simulink model "VelRefControlSim_ForThesis"  (R2016b)
settings: Solver=ode2  StartTime=0.0  StopTime=525  FixedStep=0.001  MaxStep=0.01  MinStep=0.0005  RelTol=1e-2  AbsTol=1e-3
undefined symbols (not defined in the file or in its folder): DiscIntNeverNeededParam, model_identific_dy8147ea57gM
libraries: simulink x8, powerlib_meascontrol x3, dspswit3 x1, fmu_cs_lib x1
settings Model: Creator=vamsikrishna95  LastModifiedBy=vamsikrishna95
settings SolverCC: InitialStep=0.0005  MaxConsecutiveMinStep=100  ZeroCrossAlgorithm=Adaptive

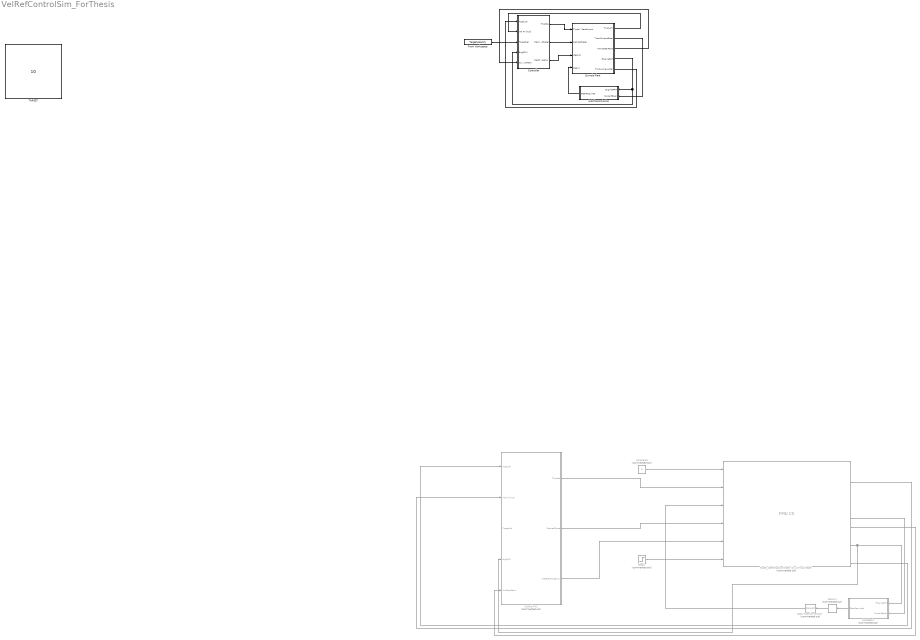
== system VelRefControlSim_ForThesis ==
  AutoGear1 : Subsystem  Commented=on
  AutoTransmission : Subsystem
  Constant1 : Constant  Commented=on  Value=0  OutDataTypeStr=Inherit: Inherit via back propagation
  Control FV2 : Subsystem  Commented=on
  Controller : Subsystem
  Data Type Conversion : DataTypeConversion  Commented=on
  Dymola Plant : Subsystem  Tag=21-Aug-2018 15:18:52#8147  LoadFcn=if exist('newDymolaGui') newDymolaGui('VelRefControlSim_TemptoDel/Dymola Plant','PostLoadNew'); else error('Dymola not installed. Must install at least the file newDymolaGui.p'); end;
      mask help:
      | Dymola block.
      | A dymola block allows acausal physical modeling.
      | See Dymola manual for usage.
      settings: CopyFcn=newDymolaGui('21-Aug-2018 15:18:52#8147','Copy');  DeleteFcn=if exist('newDymolaGui') newDymolaGui('VelRefControlSim_TemptoDel/Dymola Plant','Delete'); end;  NameChangeFcn=newDymolaGui('21-Aug-2018 15:18:52#8147','Copy');  OpenFcn=newDymolaGui('VelRefControlSim_TemptoDel/Dymola Plant','Init');
  From Workspace : FromWorkspace  VariableName=TargetVelocity  SampleTime=0
  Memory : Memory  Commented=on  X0=2  InheritSampleTime=on
  Model_Identification.Model_ID_v2.TruckModel : fmu_cs_lib/FMU CS  Description=Simulates an FMU for Co-Simulation 1.0 or Co-Simulation 2.0.  Commented=on  dummy=0
  Step1 : Step  Commented=on  Time=3  Before=1  After=0  SampleTime=0
  TARGET : Constant  Value=10  OutDataTypeStr=Inherit: Inherit via back propagation
  wires:
  AutoGear1/1(GearRequired) -> Memory/1
  Model_Identification.Model_ID_v2.TruckModel/7 -> AutoGear1/2(CurrentGear)
  Model_Identification.Model_ID_v2.TruckModel/10 -> Control FV2/4(EngRPM), AutoGear1/1(EngineRPM)
  Memory/1 -> Data Type Conversion/1
  Data Type Conversion/1 -> Model_Identification.Model_ID_v2.TruckModel/3
  Step1/1 -> Model_Identification.Model_ID_v2.TruckModel/6
  Constant1/1 -> Model_Identification.Model_ID_v2.TruckModel/1
  Controller/1(Throttle) -> Dymola Plant/1(ThrottlePedalInput)
  Controller/2(DesiredDecel) -> Dymola Plant/2(DesiredDecel)
  Controller/3(DesBrakeUrgency) -> Dymola Plant/3(Urgency)
  Control FV2/1(Throttle) -> Model_Identification.Model_ID_v2.TruckModel/2
  Control FV2/2(DesiredDecel) -> Model_Identification.Model_ID_v2.TruckModel/4
  Control FV2/3(DesBrakeUrgency) -> Model_Identification.Model_ID_v2.TruckModel/5
  Model_Identification.Model_ID_v2.TruckModel/12 -> Control FV2/1(Accel_FV)
  Model_Identification.Model_ID_v2.TruckModel/3 -> Control FV2/2(Vel FV [m/s])
  Model_Identification.Model_ID_v2.TruckModel/8 -> Control FV2/5(CurGearRatio)
  Dymola Plant/2(TransCurrentGear) -> AutoTransmission/2(CurrentGear)
  Dymola Plant/5(Truck_Long_Accel) -> Controller/1(Accel_FV)
  Dymola Plant/4(EngineRPM) -> Controller/4(EngRPM), AutoTransmission/1(EngineRPM)
  Dymola Plant/3(TransGearRatio) -> Controller/5(CurGearRatio)
  Dymola Plant/1(Truck_dX) -> Controller/2(Vel FV [m/s])
  AutoTransmission/1(GearRequired) -> Dymola Plant/4(GearIn)
  From Workspace/1 -> Controller/3(TargetVel)

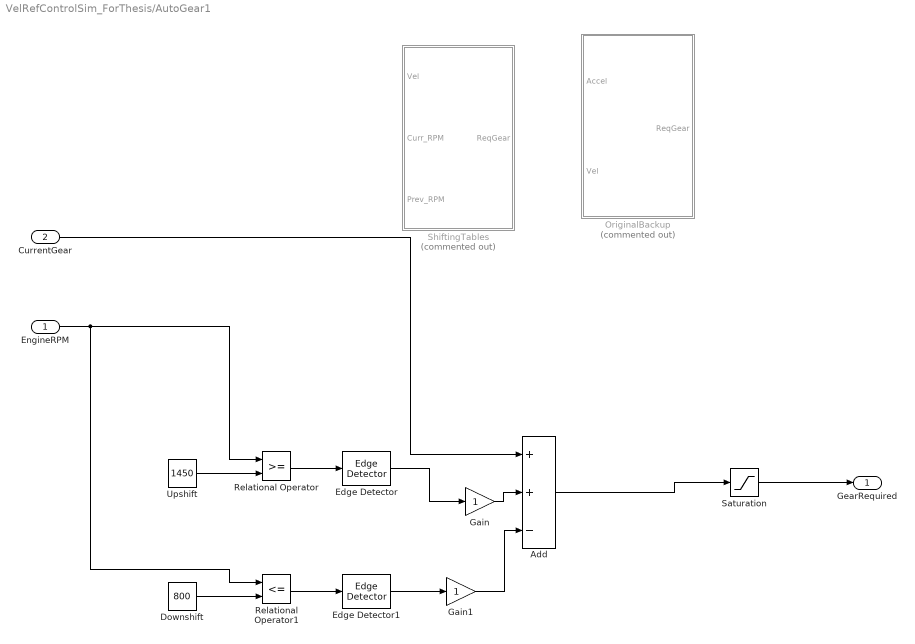
== system VelRefControlSim_ForThesis/AutoGear1 ==
  EngineRPM : Inport
  CurrentGear : Inport  Port=2
  Add : Sum  Inputs=++-
  Downshift : Constant  Value=800
  Edge Detector : powerlib_meascontrol/Logic/Edge Detector  model=Rising  ic=0  Ts=0
  Edge Detector1 : powerlib_meascontrol/Logic/Edge Detector  model=Rising  ic=0  Ts=0
  Gain : Gain
  Gain1 : Gain
  OriginalBackup : MATLAB Function  Commented=on  TreatAsAtomicUnit=on
  Relational Operator : RelationalOperator  OutDataTypeStr=boolean  RndMeth=Simplest
  Relational Operator1 : RelationalOperator  Operator=<=  OutDataTypeStr=boolean  RndMeth=Simplest
  Saturation : Saturate  UpperLimit=10  LowerLimit=0
  ShiftingTables : MATLAB Function  Commented=on  TreatAsAtomicUnit=on
  Upshift : Constant  Value=1450
  GearRequired : Outport
  wires:
  EngineRPM/1 -> Relational Operator1/1, Relational Operator/1
  Upshift/1 -> Relational Operator/2
  Downshift/1 -> Relational Operator1/2
  Relational Operator/1 -> Edge Detector/1
  Relational Operator1/1 -> Edge Detector1/1
  CurrentGear/1 -> Add/1
  Add/1 -> Saturation/1
  Edge Detector/1 -> Gain/1
  Gain/1 -> Add/2
  Edge Detector1/1 -> Gain1/1
  Gain1/1 -> Add/3
  Saturation/1 -> GearRequired/1

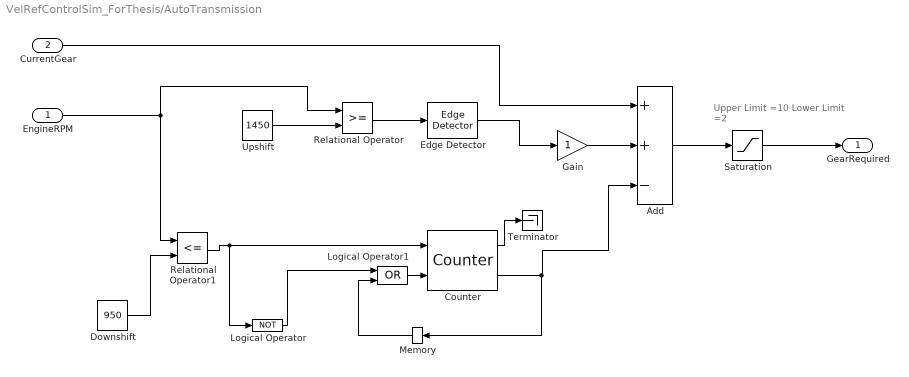
== system VelRefControlSim_ForThesis/AutoTransmission ==
  note: Upper Limit =10
      | Lower Limit =2
  EngineRPM : Inport
  CurrentGear : Inport  Port=2
  Add : Sum  Inputs=++-
  Counter : dspswit3/Counter  Direction=Up  CountEvent=Non-zero sample  CounterSize=32 bits  MaxCount=250  InitialCount=0  Output=Count and Hit  HitValue=500  ResetInput=on  SamplesPerFrame=1  Ts=1  CntDtype=double  HitDtype=Boolean
  Downshift : Constant  Value=950
  Edge Detector : powerlib_meascontrol/Logic/Edge Detector  model=Rising  ic=0  Ts=0
  Gain : Gain
  Logical Operator : Logic  Operator=NOT  AllPortsSameDT=off  OutDataTypeStr=boolean
  Logical Operator1 : Logic  Operator=OR  AllPortsSameDT=off  OutDataTypeStr=boolean
  Memory : Memory
  Relational Operator : RelationalOperator  OutDataTypeStr=boolean  RndMeth=Simplest
  Relational Operator1 : RelationalOperator  Operator=<=  OutDataTypeStr=boolean  RndMeth=Simplest
  Saturation : Saturate  UpperLimit=10  LowerLimit=2
  Terminator : Terminator
  Upshift : Constant  Value=1450
  GearRequired : Outport
  wires:
  EngineRPM/1 -> Relational Operator/1, Relational Operator1/1
  Upshift/1 -> Relational Operator/2
  Downshift/1 -> Relational Operator1/2
  Relational Operator/1 -> Edge Detector/1
  Relational Operator1/1 -> Logical Operator/1, Counter/1
  CurrentGear/1 -> Add/1
  Add/1 -> Saturation/1
  Edge Detector/1 -> Gain/1
  Gain/1 -> Add/2
  Counter/2 -> Add/3, Memory/1
  Saturation/1 -> GearRequired/1
  Logical Operator/1 -> Logical Operator1/1
  Logical Operator1/1 -> Counter/2
  Memory/1 -> Logical Operator1/2
  Counter/1 -> Terminator/1

== system VelRefControlSim_ForThesis/Control FV2 ==
  Accel_FV : Inport
  Vel FV [m/s] : Inport  Port=2
  TargetVel : Inport  Port=3
  EngRPM : Inport  Port=4
  CurGearRatio : Inport  Port=5
  TAMU_LC3 : Subsystem
  Throttle : Outport
  DesiredDecel : Outport  Port=2
  DesBrakeUrgency : Outport  Port=3
  wires:
  EngRPM/1 -> TAMU_LC3/5(EngRPM1)
  Accel_FV/1 -> TAMU_LC3/1(aFV_mps2)
  TAMU_LC3/1(Throttle) -> Throttle/1
  TAMU_LC3/2(DesiredDecel) -> DesiredDecel/1
  TAMU_LC3/3(DesBrakeUrgency) -> DesBrakeUrgency/1
  CurGearRatio/1 -> TAMU_LC3/3(CurGearRatio)
  TargetVel/1 -> TAMU_LC3/4(TargetVel)
  Vel FV [m/s]/1 -> TAMU_LC3/2(vFV_mps)

== system VelRefControlSim_ForThesis/Controller ==
  Accel_FV : Inport
  Vel FV [m/s] : Inport  Port=2
  TargetVel : Inport  Port=3
  EngRPM : Inport  Port=4
  CurGearRatio : Inport  Port=5
  TAMU_LC3 : Subsystem
  Throttle : Outport
  DesiredDecel : Outport  Port=2
  DesBrakeUrgency : Outport  Port=3
  wires:
  Vel FV [m/s]/1 -> TAMU_LC3/2(Current_Velocity)
  TargetVel/1 -> TAMU_LC3/4(Target_Velocity)
  CurGearRatio/1 -> TAMU_LC3/3(CurGearRatio)
  TAMU_LC3/3(DesBrakeUrgency) -> DesBrakeUrgency/1
  TAMU_LC3/2(DesiredDeceleration) -> DesiredDecel/1
  TAMU_LC3/1(Throttle) -> Throttle/1
  Accel_FV/1 -> TAMU_LC3/1(Current_Acceleration)
  EngRPM/1 -> TAMU_LC3/5(EngineRPM)

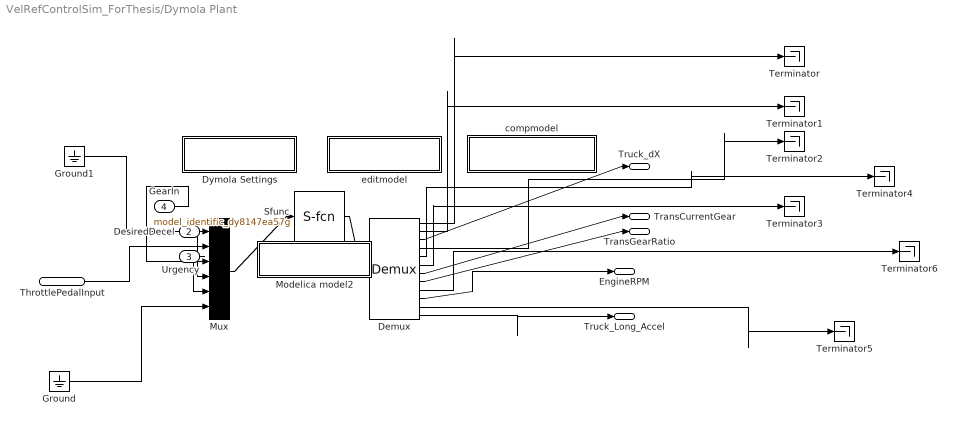
== system VelRefControlSim_ForThesis/Dymola Plant ==
  ThrottlePedalInput : Inport
  DesiredDecel : Inport  Port=2
  Urgency : Inport  Port=3
  GearIn : Inport  Port=4
  Demux : Demux  Outputs=[1;1;1;1;1;1;1;1;1;1;1;1]
  Dymola Settings : Subsystem  mask{ModelName=Model_Identification.Model_ID_v2.TruckModel, MoFileName=C:/Users/vamsikrishna95/OneDrive - Texas A&M University/MS Research/Dymola/Model Identification/Model_Identification.mo, dSpace=, BusConnector=[], ResultFile=[], ResultFileOnline=[], ResultDt=[], Libs=:HydraulicsLib:, bigobj=1, ImportFolder=[], guimode=[], ModelName2=[], forRuntime=[], MEXLoad=[], omitDescription=[]}
      mask prompts: ModelName "Name of Dymola model"; MoFileName "File Name (including .mo)"; ResultFile "Create Result"; ResultFileOnline "Load result"; ResultDt "Result min dt"; Libs "Used Libraries"; bigobj "Compiler flag /bigobj"; ImportFolder "Import folder"; guimode "GUI mode flag"; ModelName2 "Model name for import mode"; forRuntime "Runtime export"; MEXLoad "Compiled S-function"; omitDescription "Omit description strings"
      mask Display: disp('Dymola Settings');
  Ground : Ground
  Ground1 : Ground
  Modelica model2 : Subsystem
      mask Display: disp('Change parameters');
  Mux : Mux  Inputs=[1;1;1;1;1;1]
  Sfunc : S-Function  Tag=8147ea57g  FunctionName=model_identific_dy8147ea57g  Parameters=[model_identific_dy8147ea57gM.pV],[model_identific_dy8147ea57gM.x0V]  PortCounts=[1;1]  SFunctionDeploymentMode=off  EnableBusSupport=off
      mask Display: image(imread('Dymola.bmp'))
  Terminator{,1..6} (7 alike) : Terminator
  compmodel : Subsystem
      settings: OpenFcn=compileModelica('VelRefControlSim_TemptoDel/Dymola Plant');
      mask Display: disp('Compile Modelica model');
  editmodel : Subsystem
      settings: OpenFcn=editModelica('VelRefControlSim_TemptoDel/Dymola Plant');
      mask Display: disp('Edit Modelica model');
  Truck_dX : Outport
  TransCurrentGear : Outport  Port=2
  TransGearRatio : Outport  Port=3
  EngineRPM : Outport  Port=4
  Truck_Long_Accel : Outport  Port=5
  wires:
  Sfunc/1 -> Demux/1
  Demux/1 -> Terminator/1
  Demux/2 -> Terminator1/1
  Demux/3 -> Truck_dX/1
  Demux/4 -> Terminator2/1
  Demux/5 -> Terminator4/1
  Demux/6 -> Terminator3/1
  Demux/7 -> TransCurrentGear/1
  Demux/8 -> TransGearRatio/1
  Demux/9 -> Terminator6/1
  Demux/10 -> EngineRPM/1
  Demux/11 -> Terminator5/1
  Demux/12 -> Truck_Long_Accel/1
  Mux/1 -> Sfunc/1
  Ground1/1 -> Mux/1
  ThrottlePedalInput/1 -> Mux/2
  GearIn/1 -> Mux/3
  DesiredDecel/1 -> Mux/4
  Urgency/1 -> Mux/5
  Ground/1 -> Mux/6

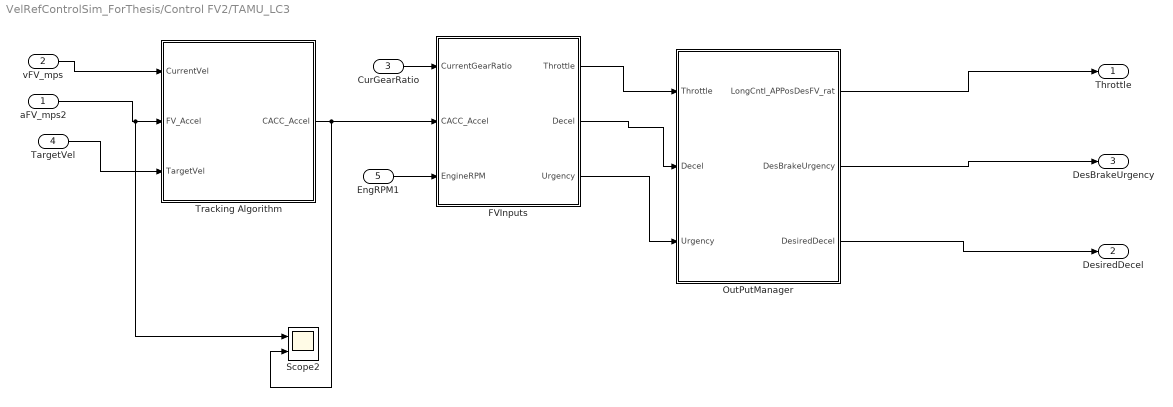
== system VelRefControlSim_ForThesis/Control FV2/TAMU_LC3 ==
  aFV_mps2 : Inport
  vFV_mps : Inport  Port=2
  CurGearRatio : Inport  Port=3
  TargetVel : Inport  Port=4
  EngRPM1 : Inport  Port=5
  FVInputs : Subsystem
  OutPutManager : Subsystem
  Scope2 : Scope  NumInputPorts=2
  Tracking Algorithm : Subsystem
  Throttle : Outport
  DesiredDecel : Outport  Port=2
  DesBrakeUrgency : Outport  Port=3
  wires:
  Tracking Algorithm/1(CACC_Accel) -> Scope2/2, FVInputs/2(CACC_Accel)
  vFV_mps/1 -> Tracking Algorithm/1(CurrentVel)
  EngRPM1/1 -> FVInputs/3(EngineRPM)
  CurGearRatio/1 -> FVInputs/1(CurrentGearRatio)
  aFV_mps2/1 -> Scope2/1, Tracking Algorithm/2(FV_Accel)
  FVInputs/1(Throttle) -> OutPutManager/1(Throttle)
  FVInputs/3(Urgency) -> OutPutManager/3(Urgency)
  OutPutManager/1(LongCntl_APPosDesFV_rat) -> Throttle/1
  OutPutManager/2(DesBrakeUrgency) -> DesBrakeUrgency/1
  OutPutManager/3(DesiredDecel) -> DesiredDecel/1
  FVInputs/2(Decel) -> OutPutManager/2(Decel)
  TargetVel/1 -> Tracking Algorithm/3(TargetVel)

== system VelRefControlSim_ForThesis/Controller/TAMU_LC3 ==
  Current_Acceleration : Inport
  Current_Velocity : Inport  Port=2
  CurGearRatio : Inport  Port=3
  Target_Velocity : Inport  Port=4
  EngineRPM : Inport  Port=5
  OutPutManager : Subsystem
  Plant Inversion : Subsystem
  Tracking Algorithm : Subsystem
  Throttle : Outport
  DesiredDeceleration : Outport  Port=2
  DesBrakeUrgency : Outport  Port=3
  wires:
  Tracking Algorithm/1(Target_Accel) -> Plant Inversion/3(Target_Accel)
  Current_Velocity/1 -> Plant Inversion/2(CurrentVelocity), Tracking Algorithm/1(CurrentVel)
  EngineRPM/1 -> Plant Inversion/4(EngineRPM)
  CurGearRatio/1 -> Plant Inversion/1(CurrentGearRatio)
  Current_Acceleration/1 -> Tracking Algorithm/2(FV_Accel)
  Plant Inversion/1(Throttle) -> OutPutManager/1(Throttle)
  Plant Inversion/3(Urgency) -> OutPutManager/3(Urgency)
  OutPutManager/1(ThrottlePosition) -> Throttle/1
  OutPutManager/2(DesBrakeUrgency) -> DesBrakeUrgency/1
  OutPutManager/3(DesiredDecel) -> DesiredDeceleration/1
  Plant Inversion/2(Decel) -> OutPutManager/2(Decel)
  Target_Velocity/1 -> Tracking Algorithm/3(TargetVel)

== system VelRefControlSim_ForThesis/Dymola Plant/Dymola Settings ==

== system VelRefControlSim_ForThesis/Dymola Plant/Modelica model2 ==

== system VelRefControlSim_ForThesis/Dymola Plant/compmodel ==

== system VelRefControlSim_ForThesis/Dymola Plant/editmodel ==

== system VelRefControlSim_ForThesis/Control FV2/TAMU_LC3/FVInputs ==
  CurrentGearRatio : Inport
  CACC_Accel : Inport  Port=2
  EngineRPM : Inport  Port=3
  CalculateCommands : Subsystem
  Vel1 : InportShadow
  Throttle : Outport
  Decel : Outport  Port=2
  Urgency : Outport  Port=3
  wires:
  CalculateCommands/1(Throttle) -> Throttle/1
  CalculateCommands/3(Urgency) -> Urgency/1
  CalculateCommands/2(Decel) -> Decel/1
  CACC_Accel/1 -> CalculateCommands/1(AccelerationCommand)
  Vel1/1 -> CalculateCommands/3(Vel)
  EngineRPM/1 -> CalculateCommands/4(CurrentRPM)
  CurrentGearRatio/1 -> CalculateCommands/2(GearRatio)

== system VelRefControlSim_ForThesis/Control FV2/TAMU_LC3/OutPutManager ==
  Throttle : Inport
  Decel : Inport  Port=2
  Urgency : Inport  Port=3
  LongCntl_APPosDesFV_rat : Outport
  DesBrakeUrgency : Outport  Port=2
  DesiredDecel : Outport  Port=3
  wires:
  Throttle/1 -> LongCntl_APPosDesFV_rat/1
  Urgency/1 -> DesBrakeUrgency/1
  Decel/1 -> DesiredDecel/1

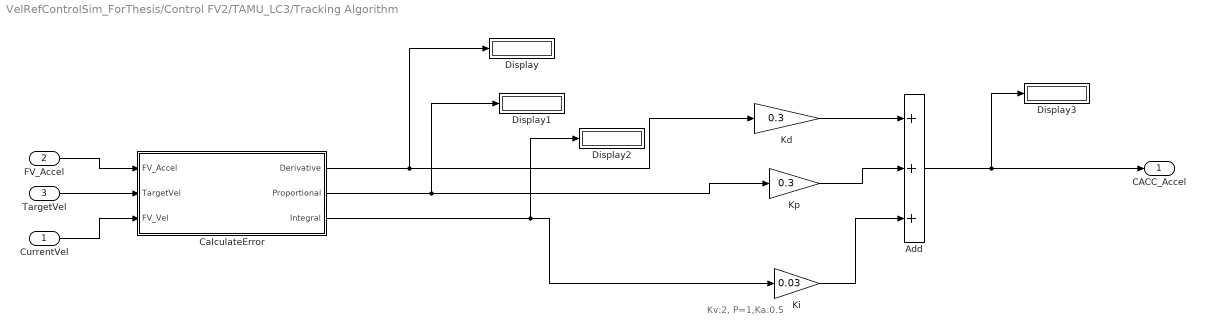
== system VelRefControlSim_ForThesis/Control FV2/TAMU_LC3/Tracking Algorithm ==
  note: Kv:2, P=1,Ka:0.5
  CurrentVel : Inport
  FV_Accel : Inport  Port=2
  TargetVel : Inport  Port=3
  Add : Sum  Inputs=+++
  CalculateError : Subsystem
  Display{,1..3} (4 alike) : Display
  Kd : Gain  Gain=0.3
  Ki : Gain  Gain=0.03
  Kp : Gain  Gain=0.3
  CACC_Accel : Outport
  wires:
  Add/1 -> Display3/1, CACC_Accel/1
  Ki/1 -> Add/3
  Kp/1 -> Add/2
  Kd/1 -> Add/1
  TargetVel/1 -> CalculateError/2(TargetVel)
  CalculateError/3(Integral) -> Display2/1, Ki/1
  CalculateError/1(Derivative) -> Display/1, Kd/1
  CalculateError/2(Proportional) -> Display1/1, Kp/1
  CurrentVel/1 -> CalculateError/3(FV_Vel)
  FV_Accel/1 -> CalculateError/1(FV_Accel)

== system VelRefControlSim_ForThesis/Controller/TAMU_LC3/OutPutManager ==
  Throttle : Inport
  Decel : Inport  Port=2
  Urgency : Inport  Port=3
  ThrottlePosition : Outport
  DesBrakeUrgency : Outport  Port=2
  DesiredDecel : Outport  Port=3
  wires:
  Throttle/1 -> ThrottlePosition/1
  Urgency/1 -> DesBrakeUrgency/1
  Decel/1 -> DesiredDecel/1

== system VelRefControlSim_ForThesis/Controller/TAMU_LC3/Plant Inversion ==
  CurrentGearRatio : Inport
  CurrentVelocity : Inport  Port=2
  Target_Accel : Inport  Port=3
  EngineRPM : Inport  Port=4
  CalculateCommands : Subsystem
  Throttle : Outport
  Decel : Outport  Port=2
  Urgency : Outport  Port=3
  wires:
  CalculateCommands/1(Throttle) -> Throttle/1
  CalculateCommands/3(Urgency) -> Urgency/1
  CalculateCommands/2(Decel) -> Decel/1
  Target_Accel/1 -> CalculateCommands/1(Target_Accel)
  CurrentVelocity/1 -> CalculateCommands/3(Vel)
  EngineRPM/1 -> CalculateCommands/4(CurrentRPM)
  CurrentGearRatio/1 -> CalculateCommands/2(GearRatio)

== system VelRefControlSim_ForThesis/Controller/TAMU_LC3/Tracking Algorithm ==
  CurrentVel : Inport
  FV_Accel : Inport  Port=2
  TargetVel : Inport  Port=3
  Add : Sum  Inputs=+++
  CalculateError : Subsystem
  Kd : Gain  Gain=0.3
  Ki : Gain  Gain=0.03
  Kp : Gain  Gain=1.5
  Target_Accel : Outport
  wires:
  Add/1 -> Target_Accel/1
  Ki/1 -> Add/3
  Kp/1 -> Add/2
  Kd/1 -> Add/1
  TargetVel/1 -> CalculateError/2(TargetVel)
  CalculateError/3(Integral) -> Ki/1
  CalculateError/1(Derivative) -> Kd/1
  CalculateError/2(Proportional) -> Kp/1
  CurrentVel/1 -> CalculateError/3(FV_Vel)
  FV_Accel/1 -> CalculateError/1(FV_Accel)

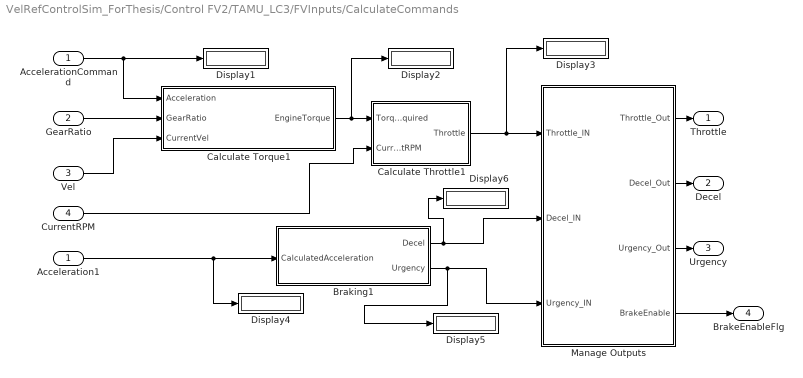
== system VelRefControlSim_ForThesis/Control FV2/TAMU_LC3/FVInputs/CalculateCommands ==
  AccelerationCommand : Inport
  GearRatio : Inport  Port=2
  Vel : Inport  Port=3
  CurrentRPM : Inport  Port=4
  Acceleration1 : InportShadow
  Braking1 : Subsystem
  Calculate Throttle1 : Subsystem
  Calculate Torque1 : Subsystem
  Display{1..6} (6 alike) : Display
  Manage Outputs : Subsystem
  Throttle : Outport
  Decel : Outport  Port=2
  Urgency : Outport  Port=3
  BrakeEnableFlg : Outport  Port=4
  wires:
  Vel/1 -> Calculate Torque1/3(CurrentVel)
  Manage Outputs/1(Throttle_Out) -> Throttle/1
  Manage Outputs/2(Decel_Out) -> Decel/1
  Manage Outputs/3(Urgency_Out) -> Urgency/1
  Manage Outputs/4(BrakeEnable) -> BrakeEnableFlg/1
  Calculate Torque1/1(EngineTorque) -> Display2/1, Calculate Throttle1/1(TorqueRequired)
  Braking1/1(Decel) -> Display6/1, Manage Outputs/2(Decel_IN)
  Braking1/2(Urgency) -> Display5/1, Manage Outputs/3(Urgency_IN)
  Calculate Throttle1/1(Throttle) -> Display3/1, Manage Outputs/1(Throttle_IN)
  AccelerationCommand/1 -> Display1/1, Calculate Torque1/1(Acceleration)
  GearRatio/1 -> Calculate Torque1/2(GearRatio)
  Acceleration1/1 -> Display4/1, Braking1/1(CalculatedAcceleration)
  CurrentRPM/1 -> Calculate Throttle1/2(CurrentRPM)

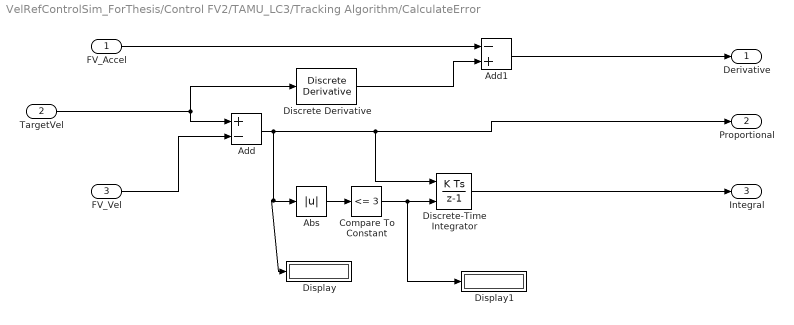
== system VelRefControlSim_ForThesis/Control FV2/TAMU_LC3/Tracking Algorithm/CalculateError ==
  FV_Accel : Inport
  TargetVel : Inport  Port=2
  FV_Vel : Inport  Port=3
  Abs : Abs
  Add : Sum  Inputs=+-
  Add1 : Sum  Inputs=-+
  Compare To Constant : simulink/Logic and Bit Operations/Compare To Constant  relop=<=  const=3  OutDataTypeStr=boolean
  Discrete Derivative : simulink/Discrete/Discrete Derivative  gainval=1.0  ICPrevScaledInput=0.0  OutMin=[]  OutMax=[]  OutDataType=fixdt(1, 16)  OutScaling=2^-10  DoSatur=off
  Discrete-Time Integrator : DiscreteIntegrator  ExternalReset=either  InitialConditionSetting=State (most efficient)  SampleTime=-1  ICPrevOutput=DiscIntNeverNeededParam  ICPrevScaledInput=DiscIntNeverNeededParam
  Display : Display
  Display1 : Display
  Derivative : Outport
  Proportional : Outport  Port=2
  Integral : Outport  Port=3
  wires:
  FV_Vel/1 -> Add/2
  Add/1 -> Display/1, Abs/1, Discrete-Time Integrator/1, Proportional/1
  Discrete-Time Integrator/1 -> Integral/1
  Compare To Constant/1 -> Display1/1, Discrete-Time Integrator/2
  Abs/1 -> Compare To Constant/1
  FV_Accel/1 -> Add1/1
  Add1/1 -> Derivative/1
  Discrete Derivative/1 -> Add1/2
  TargetVel/1 -> Discrete Derivative/1, Add/1

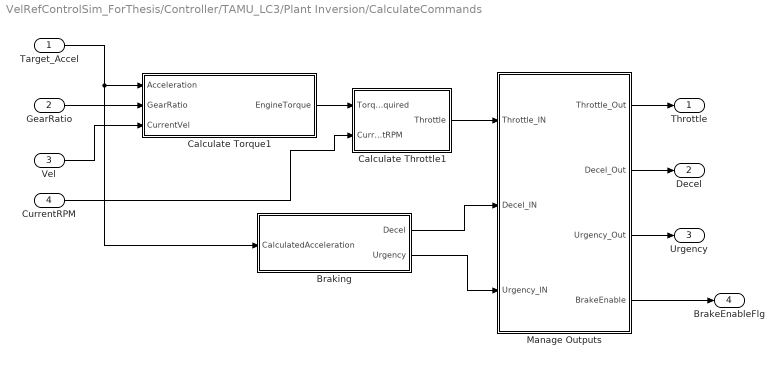
== system VelRefControlSim_ForThesis/Controller/TAMU_LC3/Plant Inversion/CalculateCommands ==
  Target_Accel : Inport
  GearRatio : Inport  Port=2
  Vel : Inport  Port=3
  CurrentRPM : Inport  Port=4
  Braking : Subsystem
  Calculate Throttle1 : Subsystem
  Calculate Torque1 : Subsystem
  Manage Outputs : Subsystem
  Throttle : Outport
  Decel : Outport  Port=2
  Urgency : Outport  Port=3
  BrakeEnableFlg : Outport  Port=4
  wires:
  Vel/1 -> Calculate Torque1/3(CurrentVel)
  Manage Outputs/1(Throttle_Out) -> Throttle/1
  Manage Outputs/2(Decel_Out) -> Decel/1
  Manage Outputs/3(Urgency_Out) -> Urgency/1
  Manage Outputs/4(BrakeEnable) -> BrakeEnableFlg/1
  Calculate Torque1/1(EngineTorque) -> Calculate Throttle1/1(TorqueRequired)
  Braking/1(Decel) -> Manage Outputs/2(Decel_IN)
  Braking/2(Urgency) -> Manage Outputs/3(Urgency_IN)
  Calculate Throttle1/1(Throttle) -> Manage Outputs/1(Throttle_IN)
  Target_Accel/1 -> Braking/1(CalculatedAcceleration), Calculate Torque1/1(Acceleration)
  GearRatio/1 -> Calculate Torque1/2(GearRatio)
  CurrentRPM/1 -> Calculate Throttle1/2(CurrentRPM)

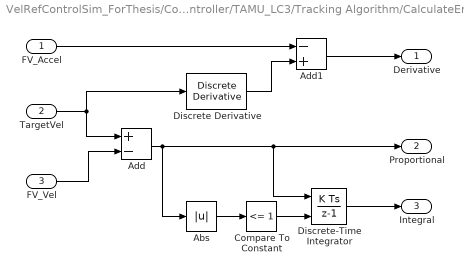
== system VelRefControlSim_ForThesis/Controller/TAMU_LC3/Tracking Algorithm/CalculateError ==
  FV_Accel : Inport
  TargetVel : Inport  Port=2
  FV_Vel : Inport  Port=3
  Abs : Abs
  Add : Sum  Inputs=+-
  Add1 : Sum  Inputs=-+
  Compare To Constant : simulink/Logic and Bit Operations/Compare To Constant  relop=<=  const=1  OutDataTypeStr=boolean
  Discrete Derivative : simulink/Discrete/Discrete Derivative  gainval=1.0  ICPrevScaledInput=0.0  OutMin=[]  OutMax=[]  OutDataType=fixdt(1, 16)  OutScaling=2^-10  DoSatur=off
  Discrete-Time Integrator : DiscreteIntegrator  ExternalReset=either  InitialConditionSetting=State (most efficient)  SampleTime=-1  ICPrevOutput=DiscIntNeverNeededParam  ICPrevScaledInput=DiscIntNeverNeededParam
  Derivative : Outport
  Proportional : Outport  Port=2
  Integral : Outport  Port=3
  wires:
  FV_Vel/1 -> Add/2
  Add/1 -> Discrete-Time Integrator/1, Proportional/1, Abs/1
  Discrete-Time Integrator/1 -> Integral/1
  Compare To Constant/1 -> Discrete-Time Integrator/2
  Abs/1 -> Compare To Constant/1
  FV_Accel/1 -> Add1/1
  Add1/1 -> Derivative/1
  Discrete Derivative/1 -> Add1/2
  TargetVel/1 -> Discrete Derivative/1, Add/1

== system VelRefControlSim_ForThesis/Control FV2/TAMU_LC3/FVInputs/CalculateCommands/Braking1 ==
  note: VVK: Urgency is always 50. Desired Deceleration is directly supplied if negetive in sign
  CalculatedAcceleration : Inport
  BrakeGain : Gain
  Constant1 : Constant  Value=0
  Product : Product
  Relational Operator : RelationalOperator  Operator=<=  OutDataTypeStr=boolean  RndMeth=Simplest
  UrgencyInput : Constant  Value=50
  Decel : Outport
  Urgency : Outport  Port=2
  wires:
  Relational Operator/1 -> Product/2
  Constant1/1 -> Relational Operator/2
  UrgencyInput/1 -> Urgency/1
  Product/1 -> BrakeGain/1
  CalculatedAcceleration/1 -> Relational Operator/1, Product/1
  BrakeGain/1 -> Decel/1  "DesiredDecel"

== system VelRefControlSim_ForThesis/Control FV2/TAMU_LC3/FVInputs/CalculateCommands/Calculate Throttle1 ==
  TorqueRequired : Inport
  CurrentRPM : Inport  Port=2
  2-D Lookup Table : Lookup_n-D  BreakpointsForDimension1=[614,780,920,1060,1200,1340,1480,1620,1760,1900]  BreakpointsForDimension2=[0,0.1,0.2,0.3,0.4,0.5,0.6,0.7,0.8,0.9,1]  Table=reshape([86.73611514,105.8405655,113.1996699,67.6591631,-58.19508728,-191.8113401,-293.2828801,-369.4632295,-429.6811752,-481.9106331,76.98368491,131.2358329,215.0818792,240.6971234,107.2585348,13.76654832,-66.37849906,-136.6523609,-188.4147634,-230.0703964,78.97660067,186.0400195,303.2239559,313.7692101,305.3571826,266.1046744,163.0011467,94.80363664,52.86622034,13.78135251,74.86631012,336.5316227,527.886412,634.6263075,794.34598,588.8393662,385.2152943,340.5948559,295.8784275,231.5493563,36.68374347,526.7430693,941.1148605,974.2037278,927.9216935,873.8393758,698.0261424,631.1730108,521.7835127,402.2858092,6.770354197,590.1855379,1125.245839,1102.847737,1134.382167,1188.884574,1143.342244,857.4068452,672.613835,524.6555484,103.1551303,590.278062,1376.620093,1457.903799,1364.105188,1264.916741,1244.794833,826.568468,712.7217089,607.4316163,492.2219427,1051.188312,1633.737735,1571.373926,1474.118512,1436.479582,1339.916646,751.7731122,578.9865072,622.5523318,1041.135563,1392.252488,1610.965726,1641.217364,1439.001055,1366.920903,965.899271,988.0607633,709.0623378,533.3993472,1593.47771,1724.886125,1811.693877,1871.009293,1707.597612,1593.086058,1526.423646,1184.232217,803.8046535,453.7427334,2125.233789,2084.15899,2063.670259,2057.714438,2008.990136,1903.282745,1693.581693,1248.844871,831.3965021,394.0171266],10,11)  InternalRulePriority=Speed  RndMeth=Simplest  InputSameDT=on
  Memory1 : Memory  X0=600  InheritSampleTime=on
  Saturation : Saturate  UpperLimit=1900  LowerLimit=614
  ThrottleCalculation : MATLAB Function  TreatAsAtomicUnit=on
  ZGrid1 : Constant  Value=[0,0.1,0.2,0.3,0.4,0.5,0.6,0.7,0.8,0.9,1]
  Throttle : Outport
  wires:
  CurrentRPM/1 -> Memory1/1
  TorqueRequired/1 -> ThrottleCalculation/2(Trq_dmnd)
  ZGrid1/1 -> 2-D Lookup Table/2
  2-D Lookup Table/1 -> ThrottleCalculation/1(Trq_interp)
  Saturation/1 -> 2-D Lookup Table/1
  ThrottleCalculation/1(Req_Thr) -> Throttle/1
  Memory1/1 -> Saturation/1

== system VelRefControlSim_ForThesis/Control FV2/TAMU_LC3/FVInputs/CalculateCommands/Calculate Torque1 ==
  Acceleration : Inport
  GearRatio : Inport  InitFcn=CurrentGear=5;  Port=2
  CurrentVel : Inport  Port=3
  CalculateWheelTrq : Subsystem
  Divide : Product  Inputs=*//
  DrivelineRatio : Constant  Value=3.3
  Saturation : Saturate  UpperLimit=2305.5
  EngineTorque : Outport
  wires:
  Saturation/1 -> EngineTorque/1
  GearRatio/1 -> Divide/2
  Acceleration/1 -> CalculateWheelTrq/1(Accel)
  CurrentVel/1 -> CalculateWheelTrq/2(CurrentVel)
  Divide/1 -> Saturation/1
  DrivelineRatio/1 -> Divide/3
  CalculateWheelTrq/1(WheelTrq) -> Divide/1

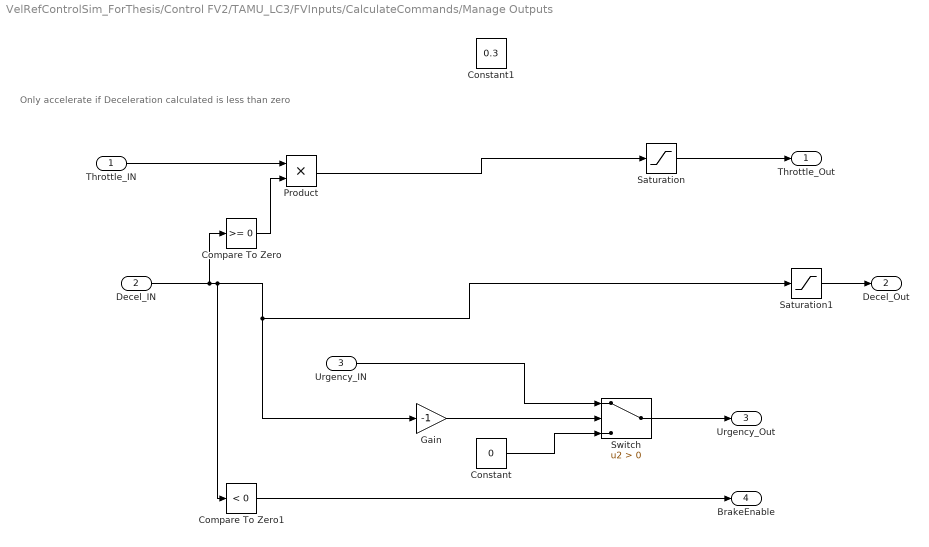
== system VelRefControlSim_ForThesis/Control FV2/TAMU_LC3/FVInputs/CalculateCommands/Manage Outputs ==
  note: Only accelerate if Deceleration calculated is less than zero
  Throttle_IN : Inport
  Decel_IN : Inport  Port=2
  Urgency_IN : Inport  Port=3
  Compare To Zero : simulink/Logic and Bit Operations/Compare To Zero  relop=>=  OutDataTypeStr=boolean
  Compare To Zero1 : simulink/Logic and Bit Operations/Compare To Zero  relop=<  OutDataTypeStr=boolean
  Constant : Constant  Value=0
  Constant1 : Constant  Value=0.3
  Gain : Gain  Gain=-1
  Product : Product
  Saturation : Saturate  UpperLimit=1  LowerLimit=0
  Saturation1 : Saturate  UpperLimit=0  LowerLimit=-6
  Switch : Switch  Criteria=u2 > Threshold
  Throttle_Out : Outport
  Decel_Out : Outport  Port=2
  Urgency_Out : Outport  Port=3
  BrakeEnable : Outport  Port=4
  wires:
  Compare To Zero/1 -> Product/2
  Saturation1/1 -> Decel_Out/1
  Compare To Zero1/1 -> BrakeEnable/1
  Switch/1 -> Urgency_Out/1
  Gain/1 -> Switch/2
  Urgency_IN/1 -> Switch/1
  Constant/1 -> Switch/3
  Product/1 -> Saturation/1
  Throttle_IN/1 -> Product/1
  Saturation/1 -> Throttle_Out/1
  Decel_IN/1 -> Compare To Zero1/1, Saturation1/1, Gain/1, Compare To Zero/1

== system VelRefControlSim_ForThesis/Controller/TAMU_LC3/Plant Inversion/CalculateCommands/Braking ==
  note: VVK: Urgency is always 50. Desired Deceleration is directly supplied if negetive in sign
  CalculatedAcceleration : Inport
  BrakeGain : Gain
  Constant1 : Constant  Value=0
  Product : Product
  Relational Operator : RelationalOperator  Operator=<=  OutDataTypeStr=boolean  RndMeth=Simplest
  UrgencyInput : Constant  Value=50
  Decel : Outport
  Urgency : Outport  Port=2
  wires:
  Relational Operator/1 -> Product/2
  Constant1/1 -> Relational Operator/2
  UrgencyInput/1 -> Urgency/1
  Product/1 -> BrakeGain/1
  CalculatedAcceleration/1 -> Relational Operator/1, Product/1
  BrakeGain/1 -> Decel/1  "DesiredDecel"

== system VelRefControlSim_ForThesis/Controller/TAMU_LC3/Plant Inversion/CalculateCommands/Calculate Throttle1 ==
  note: ZGrid=[0,0.1,0.2,0.3,0.4,0.5,0.6,0.7,0.8,0.9,1]
  TorqueRequired : Inport
  CurrentRPM : Inport  Port=2
  2-D Lookup Table : Lookup_n-D  BreakpointsForDimension1=[614,780,920,1060,1200,1340,1480,1620,1760,1900]  BreakpointsForDimension2=[0,0.1,0.2,0.3,0.4,0.5,0.6,0.7,0.8,0.9,1]  Table=reshape([86.73611514,105.8405655,113.1996699,67.6591631,-58.19508728,-191.8113401,-293.2828801,-369.4632295,-429.6811752,-481.9106331,76.98368491,131.2358329,215.0818792,240.6971234,107.2585348,13.76654832,-66.37849906,-136.6523609,-188.4147634,-230.0703964,78.97660067,186.0400195,303.2239559,313.7692101,305.3571826,266.1046744,163.0011467,94.80363664,52.86622034,13.78135251,74.86631012,336.5316227,527.886412,634.6263075,794.34598,588.8393662,385.2152943,340.5948559,295.8784275,231.5493563,36.68374347,526.7430693,941.1148605,974.2037278,927.9216935,873.8393758,698.0261424,631.1730108,521.7835127,402.2858092,6.770354197,590.1855379,1125.245839,1102.847737,1134.382167,1188.884574,1143.342244,857.4068452,672.613835,524.6555484,103.1551303,590.278062,1376.620093,1457.903799,1364.105188,1264.916741,1244.794833,826.568468,712.7217089,607.4316163,492.2219427,1051.188312,1633.737735,1571.373926,1474.118512,1436.479582,1339.916646,751.7731122,578.9865072,622.5523318,1041.135563,1392.252488,1610.965726,1641.217364,1439.001055,1366.920903,965.899271,988.0607633,709.0623378,533.3993472,1593.47771,1724.886125,1811.693877,1871.009293,1707.597612,1593.086058,1526.423646,1184.232217,803.8046535,453.7427334,2125.233789,2084.15899,2063.670259,2057.714438,2008.990136,1903.282745,1693.581693,1248.844871,831.3965021,394.0171266],10,11)  InternalRulePriority=Speed  RndMeth=Simplest  InputSameDT=on
  Memory : Memory  X0=600  InheritSampleTime=on
  Saturation : Saturate  UpperLimit=1900  LowerLimit=614
  ThrottleCalculation : MATLAB Function  TreatAsAtomicUnit=on
  ZGrid : Constant  Value=[0,0.1,0.2,0.3,0.4,0.5,0.6,0.7,0.8,0.9,1]
  Throttle : Outport
  wires:
  CurrentRPM/1 -> Memory/1
  TorqueRequired/1 -> ThrottleCalculation/2(Torque_dmnd)
  ZGrid/1 -> 2-D Lookup Table/2
  2-D Lookup Table/1 -> ThrottleCalculation/1(Torque_interp)
  Saturation/1 -> 2-D Lookup Table/1
  ThrottleCalculation/1(Req_Throttle) -> Throttle/1
  Memory/1 -> Saturation/1

== system VelRefControlSim_ForThesis/Controller/TAMU_LC3/Plant Inversion/CalculateCommands/Calculate Torque1 ==
  Acceleration : Inport
  GearRatio : Inport  InitFcn=CurrentGear=5;  Port=2
  CurrentVel : Inport  Port=3
  CalculateWheelTorque : Subsystem
  Divide : Product  Inputs=*//
  DrivelineRatio : Constant  Value=3.39
  Saturation : Saturate  UpperLimit=2305.5
  EngineTorque : Outport
  wires:
  Saturation/1 -> EngineTorque/1
  GearRatio/1 -> Divide/2
  Acceleration/1 -> CalculateWheelTorque/1(Accel)
  CurrentVel/1 -> CalculateWheelTorque/2(CurrentVel)
  Divide/1 -> Saturation/1
  DrivelineRatio/1 -> Divide/3
  CalculateWheelTorque/1(WheelTorque) -> Divide/1

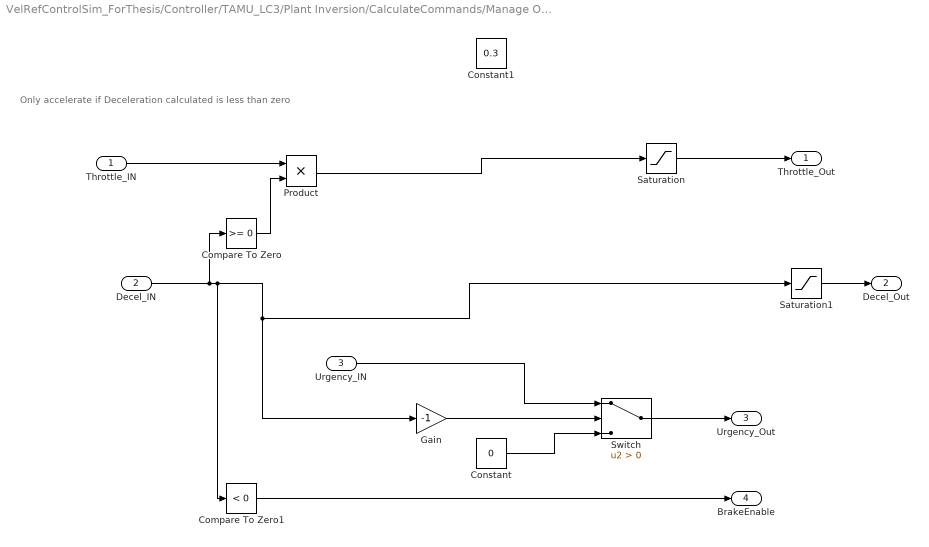
== system VelRefControlSim_ForThesis/Controller/TAMU_LC3/Plant Inversion/CalculateCommands/Manage Outputs ==
  note: Only accelerate if Deceleration calculated is less than zero
  Throttle_IN : Inport
  Decel_IN : Inport  Port=2
  Urgency_IN : Inport  Port=3
  Compare To Zero : simulink/Logic and Bit Operations/Compare To Zero  relop=>=  OutDataTypeStr=boolean
  Compare To Zero1 : simulink/Logic and Bit Operations/Compare To Zero  relop=<  OutDataTypeStr=boolean
  Constant : Constant  Value=0
  Constant1 : Constant  Value=0.3
  Gain : Gain  Gain=-1
  Product : Product
  Saturation : Saturate  UpperLimit=1  LowerLimit=0
  Saturation1 : Saturate  UpperLimit=0  LowerLimit=-6
  Switch : Switch  Criteria=u2 > Threshold
  Throttle_Out : Outport
  Decel_Out : Outport  Port=2
  Urgency_Out : Outport  Port=3
  BrakeEnable : Outport  Port=4
  wires:
  Compare To Zero/1 -> Product/2
  Saturation1/1 -> Decel_Out/1
  Compare To Zero1/1 -> BrakeEnable/1
  Switch/1 -> Urgency_Out/1
  Gain/1 -> Switch/2
  Urgency_IN/1 -> Switch/1
  Constant/1 -> Switch/3
  Product/1 -> Saturation/1
  Throttle_IN/1 -> Product/1
  Saturation/1 -> Throttle_Out/1
  Decel_IN/1 -> Compare To Zero1/1, Saturation1/1, Gain/1, Compare To Zero/1

== system VelRefControlSim_ForThesis/Control FV2/TAMU_LC3/FVInputs/CalculateCommands/Calculate Torque1/CalculateWheelTrq ==
  Accel : Inport
  CurrentVel : Inport  Port=2
  AeroDrag : Subsystem
  Combined Mass : Constant  Value=24000
  GradientResistance : Subsystem
  NetForceRequired : Sum  Inputs=++++
  Product : Product
  Product1 : Product
  RollingResistance : Subsystem
  WheelRadius : Constant  Value=0.5377
  WheelTrq : Outport
  wires:
  GradientResistance/1(GradientForce) -> NetForceRequired/4
  RollingResistance/1(RollingForce) -> NetForceRequired/3
  CurrentVel/1 -> AeroDrag/1(Vel)
  Product1/1 -> NetForceRequired/1
  Combined Mass/1 -> Product1/2
  Accel/1 -> Product1/1
  NetForceRequired/1 -> Product/1
  WheelRadius/1 -> Product/2
  Product/1 -> WheelTrq/1
  AeroDrag/1(DragForce) -> NetForceRequired/2

== system VelRefControlSim_ForThesis/Controller/TAMU_LC3/Plant Inversion/CalculateCommands/Calculate Torque1/CalculateWheelTorque ==
  Accel : Inport
  CurrentVel : Inport  Port=2
  AeroDrag : Subsystem
  Combined Mass : Constant  Value=24000
  GradientResistance : Subsystem
  NetForceRequired : Sum  Inputs=++++
  Product : Product
  Product1 : Product
  RollingResistance : Subsystem
  WheelRadius : Constant  Value=0.5377
  WheelTorque : Outport
  wires:
  GradientResistance/1(GradientForce) -> NetForceRequired/4
  RollingResistance/1(RollingForce) -> NetForceRequired/3
  CurrentVel/1 -> AeroDrag/1(Vel)
  Product1/1 -> NetForceRequired/1
  Combined Mass/1 -> Product1/2
  Accel/1 -> Product1/1
  NetForceRequired/1 -> Product/1
  WheelRadius/1 -> Product/2
  Product/1 -> WheelTorque/1
  AeroDrag/1(DragForce) -> NetForceRequired/2

== system VelRefControlSim_ForThesis/Control FV2/TAMU_LC3/FVInputs/CalculateCommands/Calculate Torque1/CalculateWheelTrq/AeroDrag ==
  Vel : Inport
  DragCoeff : Gain  Gain=0.6
  FrontalArea : Gain  Gain=7.8
  Gain : Gain  Gain=0.5
  Math Function : Math  Operator=square  SaturateOnIntegerOverflow=on
  Rho_air : Gain  Gain=1.225
  DragForce : Outport
  wires:
  DragCoeff/1 -> DragForce/1
  FrontalArea/1 -> DragCoeff/1
  Rho_air/1 -> FrontalArea/1
  Gain/1 -> Rho_air/1
  Math Function/1 -> Gain/1
  Vel/1 -> Math Function/1

== system VelRefControlSim_ForThesis/Control FV2/TAMU_LC3/FVInputs/CalculateCommands/Calculate Torque1/CalculateWheelTrq/GradientResistance ==
  note: Gradient can be calculated from IMU when installed
  Combined Mass1 : Constant  Value=24000
  Gain1 : Gain  Gain=9.81
  Gradient : Constant  Value=0
  Product : Product
  GradientForce : Outport
  wires:
  Combined Mass1/1 -> Gain1/1
  Gradient/1 -> Product/2
  Gain1/1 -> Product/1
  Product/1 -> GradientForce/1

== system VelRefControlSim_ForThesis/Control FV2/TAMU_LC3/FVInputs/CalculateCommands/Calculate Torque1/CalculateWheelTrq/RollingResistance ==
  Combined Mass1 : Constant  Value=24000
  Constant : Constant  Value=0
  Gain1 : Gain  Gain=9.81
  Product : Product
  RollingForce : Outport
  wires:
  Product/1 -> RollingForce/1
  Gain1/1 -> Product/1
  Constant/1 -> Product/2
  Combined Mass1/1 -> Gain1/1

== system VelRefControlSim_ForThesis/Controller/TAMU_LC3/Plant Inversion/CalculateCommands/Calculate Torque1/CalculateWheelTorque/AeroDrag ==
  Vel : Inport
  DragCoeff : Gain  Gain=0.6
  FrontalArea : Gain  Gain=7.8
  Gain : Gain  Gain=0.5
  Math Function : Math  Operator=square  SaturateOnIntegerOverflow=on
  Rho_air : Gain  Gain=1.225
  DragForce : Outport
  wires:
  DragCoeff/1 -> DragForce/1
  FrontalArea/1 -> DragCoeff/1
  Rho_air/1 -> FrontalArea/1
  Gain/1 -> Rho_air/1
  Math Function/1 -> Gain/1
  Vel/1 -> Math Function/1

== system VelRefControlSim_ForThesis/Controller/TAMU_LC3/Plant Inversion/CalculateCommands/Calculate Torque1/CalculateWheelTorque/GradientResistance ==
  note: Gradient can be calculated from IMU when installed
  Combined Mass1 : Constant  Value=24000
  Gain1 : Gain  Gain=9.81
  Gradient : Constant  Value=0
  Product : Product
  GradientForce : Outport
  wires:
  Combined Mass1/1 -> Gain1/1
  Gradient/1 -> Product/2
  Gain1/1 -> Product/1
  Product/1 -> GradientForce/1

== system VelRefControlSim_ForThesis/Controller/TAMU_LC3/Plant Inversion/CalculateCommands/Calculate Torque1/CalculateWheelTorque/RollingResistance ==
  Combined Mass1 : Constant  Value=24000
  Constant : Constant  Value=0
  Gain1 : Gain  Gain=9.81
  Product : Product
  RollingForce : Outport
  wires:
  Product/1 -> RollingForce/1
  Gain1/1 -> Product/1
  Constant/1 -> Product/2
  Combined Mass1/1 -> Gain1/1

== matlab function VelRefControlSim_ForThesis/Control FV2/TAMU_LC3/FVInputs/CalculateCommands/Calculate Throttle1/ThrottleCalculation ==
  data: Trq_interp input; Trq_dmnd input; Req_Thr output
function Req_Thr = fcn(Trq_interp,Trq_dmnd)
Req_Thr=double(0);
Thr_table=[0,0.1,0.2,0.3,0.4,0.5,0.6,0.7,0.8,0.9,1];
%manual interp function
for idx=1:(length(Trq_interp)-1)
    lower=Trq_interp(idx);
    upper=Trq_interp(idx+1);
    if (Trq_dmnd<upper)&&(Trq_dmnd>=lower)
        % In range, interpolate linearly
         Req_Thr=0.1*((Trq_dmnd-lower)/(upper-lower))+Thr_table(idx);
         idx=(length(Trq_interp)-1); 
         break;% quit for loop 
    else
        idx=idx+1;
    end;
end;
    
MaxTorque=double(0);
MaxTorque=double(max(Trq_interp,[],1));
MinTorque=double(0);
MinTorque=double(min(Trq_interp,[],1));
if Trq_dmnd >= MaxTorque
    Req_Thr=1;
elseif Trq_dmnd <= MinTorque
    Req_Thr=0;
end
end

== matlab function VelRefControlSim_ForThesis/Controller/TAMU_LC3/Plant Inversion/CalculateCommands/Calculate Throttle1/ThrottleCalculation ==
  data: Torque_interp input; Torque_dmnd input; Req_Throttle output
function Req_Throttle = fcn(Torque_interp,Torque_dmnd)
Req_Throttle=double(0);
Thr_table=[0,0.1,0.2,0.3,0.4,0.5,0.6,0.7,0.8,0.9,1];
%manual interp function
for idx=1:(length(Torque_interp)-1)
    lower=Torque_interp(idx);
    upper=Torque_interp(idx+1);
    if (Torque_dmnd<upper)&&(Torque_dmnd>=lower)
        % In range, interpolate linearly
         Req_Throttle=0.1*((Torque_dmnd-lower)/(upper-lower))+Thr_table(idx);
         idx=(length(Torque_interp)-1); 
         break;% quit for loop 
    else
        idx=idx+1;
    end;
end;
    
MaxTorque=double(0);
MaxTorque=double(max(Torque_interp,[],1));
MinTorque=double(0);
MinTorque=double(min(Torque_interp,[],1));
if Torque_dmnd >= MaxTorque
    Req_Throttle=1;
elseif Torque_dmnd <= MinTorque
    Req_Throttle=0;
end
end

== matlab function VelRefControlSim_ForThesis/AutoGear1/OriginalBackup ==
  data: ReqGear output; Accel input; Vel input
function ReqGear = fcn(Accel,Vel)
%#codegen
if Accel<-0.5 % Downshift
    if (Vel>-1)&&(Vel<2)
        ReqGear=2;
    elseif(Vel>=2)&&(Vel<3.3)
        ReqGear=3;
    elseif (Vel>=3.3)&&(Vel<4.5)
        ReqGear=4;
    elseif (Vel>=4.5)&&(Vel<6.2)
        ReqGear=5;
    elseif (Vel>=6.2)&&(Vel<9.7)
        ReqGear=6;
    elseif (Vel>=9.7)&&(Vel<13.4)
        ReqGear=7;
    elseif (Vel>=13.4)&&(Vel<18)
        ReqGear=8;
    elseif (Vel>=18)&&(Vel<19.4)
        ReqGear=9;
    else
        ReqGear=10;
    end;
else % Upshift
    if (Vel>-1)&&(Vel<3.2)
        ReqGear=2;
    elseif(Vel>=3.2)&&(Vel<4)
        ReqGear=3;
    elseif (Vel>=4)&&(Vel<5.4)
        ReqGear=4;
    elseif (Vel>=5.4)&&(Vel<6.8)
        ReqGear=5;
    elseif (Vel>=6.8)&&(Vel<8.4)
        ReqGear=6;
    elseif (Vel>=8.4)&&(Vel<11.2)
        ReqGear=7;
    elseif (Vel>=11.2)&&(Vel<15.3)
        ReqGear=8;
    elseif (Vel>=15.3)&&(Vel<21)
        ReqGear=9;
    else
        ReqGear=10;
    end;
end;

== matlab function VelRefControlSim_ForThesis/AutoGear1/ShiftingTables ==
  data: ReqGear output; Vel input; Curr_RPM input; Prev_RPM input
function ReqGear = fcn(Vel, Curr_RPM, Prev_RPM)
%#codegen
if Prev_RPM<Curr_RPM % Downshift
    if (Vel>-1)&&(Vel<2)
        ReqGear=2;
    elseif(Vel>=2)&&(Vel<3.3)
        ReqGear=3;
    elseif (Vel>=3.3)&&(Vel<4.5)
        ReqGear=4;
    elseif (Vel>=4.5)&&(Vel<6.2)
        ReqGear=5;
    elseif (Vel>=6.2)&&(Vel<9.7)
        ReqGear=6;
    elseif (Vel>=9.7)&&(Vel<13.4)
        ReqGear=7;
    elseif (Vel>=13.4)&&(Vel<18)
        ReqGear=8;
    elseif (Vel>=18)&&(Vel<19.4)
        ReqGear=9;
    else
        ReqGear=10;
    end;
else % Upshift
    if (Vel>-1)&&(Vel<2)
        ReqGear=2;
    elseif(Vel>=2)&&(Vel<4)
        ReqGear=3;
    elseif (Vel>=4)&&(Vel<5.4)
        ReqGear=4;
    elseif (Vel>=5.4)&&(Vel<6.8)
        ReqGear=5;
    elseif (Vel>=6.8)&&(Vel<8.4)
        ReqGear=6;
    elseif (Vel>=8.4)&&(Vel<11.2)
        ReqGear=7;
    elseif (Vel>=11.2)&&(Vel<15.3)
        ReqGear=8;
    elseif (Vel>=15.3)&&(Vel<21)
        ReqGear=9;
    else
        ReqGear=10;
    end;
end;
